simulink model "Flat_Top_Sampling_EEE311L_Exp_04"  (R2025b)
settings: Solver=VariableStepAuto  StartTime=0.0  StopTime=30  RelTol=1e-3
libraries: dspsigops x2, dspfdesign x1
settings Model: Creator=fahim  LastModifiedBy=fahim

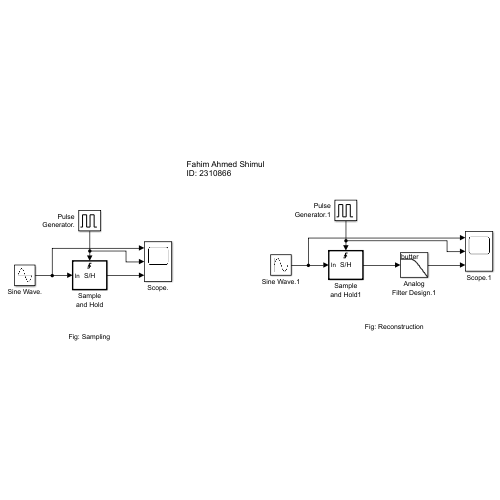
[thumbnail: Simulink's stored preview of the top-level diagram]
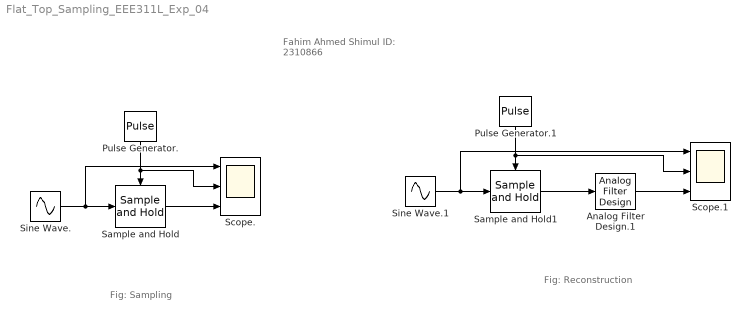
== system Flat_Top_Sampling_EEE311L_Exp_04 ==
  note: Fig: Reconstruction
  note: Fig: Sampling
  note: Fahim Ahmed Shimul
      | ID: 2310866
  Analog Filter Design.1 : dspfdesign/Analog Filter Design  method=Butterworth  filttype=Lowpass  N=2  Wlo=1  Whi=80  Rp=2  Rs=40
  Pulse Generator. : DiscretePulseGenerator  PulseType=Time based  Period=0.5  PulseWidth=50  SampleTime=0.001
  Pulse Generator.1 : DiscretePulseGenerator  PulseType=Time based  Period=0.5  PulseWidth=50  SampleTime=0.001
  Sample and Hold : dspsigops/Sample and Hold  trig=Rising edge  initCond=0  latchinput=off
  Sample and Hold1 : dspsigops/Sample and Hold  trig=Rising edge  initCond=0  latchinput=off
  Scope. : Scope  NumInputPorts=3
      settings: ActiveDisplayString=3  Title=Sampled Message ( Flat Top )  ActiveDisplayYMinimum=-1.2496758556950482  ActiveDisplayYMaximum=1.2471806357483992
  Scope.1 : Scope  NumInputPorts=3
      settings: ActiveDisplayString=3  Title=Reconstructed Signal  ActiveDisplayYMinimum=-0.888414051308079  ActiveDisplayYMaximum=0.89727831360839616
  Sine Wave. : Sin  Samples=1000  SampleTime=0
  Sine Wave.1 : Sin  Samples=1000  SampleTime=0
  wires:
  Sine Wave./1 -> Scope./1, Sample and Hold/1
  Pulse Generator./1 -> Scope./2, Sample and Hold/Trigger
  Analog Filter Design.1/1 -> Scope.1/3
  Sample and Hold1/1 -> Analog Filter Design.1/1
  Pulse Generator.1/1 -> Scope.1/2, Sample and Hold1/Trigger
  Sine Wave.1/1 -> Scope.1/1, Sample and Hold1/1
  Sample and Hold/1 -> Scope./3
